simulink model "q3c"  (R2024a)
settings: Solver=VariableStepAuto  StartTime=0.0  StopTime=10.0  RelTol=1e-3
settings Model: Creator=SHINE MOHAN S  LastModifiedBy=SHINE MOHAN S

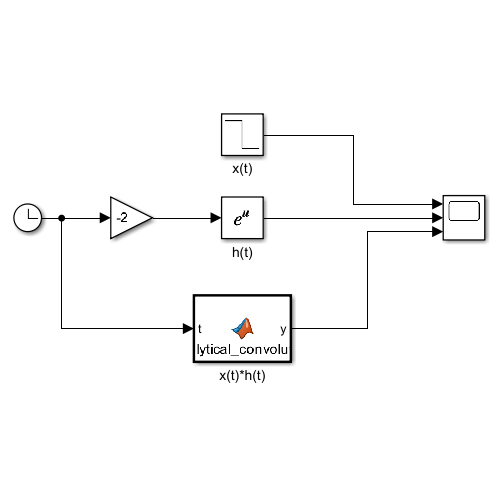
[thumbnail: Simulink's stored preview of the top-level diagram]
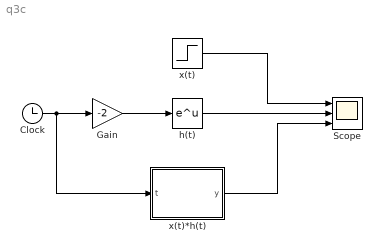
== system q3c ==
  Clock : Clock
  Gain : Gain  Gain=-2
  Scope : Scope  NumInputPorts=3
  h(t) : Math
  x(t) : Step  Time=5  Before=1  After=0  SampleTime=0
  x(t)*h(t) : MATLAB Function  TreatAsAtomicUnit=on
  wires:
  Clock/1 -> x(t)*h(t)/1(t), Gain/1
  Gain/1 -> h(t)/1
  x(t)/1 -> Scope/1
  h(t)/1 -> Scope/2
  x(t)*h(t)/1(y) -> Scope/3

== matlab function q3c/x(t)*h(t) ==
  data: t input; y output
function y = analytical_convolution(t)
    y = zeros(size(t));

    for i = 1:length(t)
        if t(i) < 0
            y(i) = 0; 
        elseif t(i) < 5
            y(i) = 0.5 * exp(-2 * t(i)) * (exp(2 * t(i)) - 1);
        else
            y(i) = (1/2) * (exp(10) - 1) * exp(-2 * t(i));
        end
    end
end
